simulink model "Quadcopter_Model_V2"  (R2022a)
settings: Solver=ode45  StartTime=0.0  StopTime=20  RelTol=1e-3
values from neighbouring files (symbols this model uses):
  disturbance = false    [Main_Script.m]
  eta = 1    [Linearize_EOM_V2.m]    (also in Properties_Quad.m)
  g = subs(f,x,x_e)    [Linearize_EOM1.m]    (also in Linearize_EOM_V2.m = 9.8; Properties_Quad.m = 9.8)
  L = (F2+F3)*dy - (F1+F4)*dy    [Linearize_EOM1.m]    (also in Linearize_EOM_V2.m = 0.114; Properties_Quad.m = 0.155)
  m = 4    [Controller_LQR.m]    (also in Linearize_EOM1.m; Linearize_EOM_V2.m; Properties_Quad.m = 1)
  noise = false    [Main_Script.m]
  sample = false    [Main_Script.m]
  T = 1-S    [Hinf_Controller_Outer.m]    (also in Properties_Quad.m = 0.01; quad_hinf.m)
  u_e = zeros(4,1)    [A_and_B_Matricies.m]    (also in Controller_LQR.m; Create_System.m; Linear_Main.mat = [2.45 2.45 2.45 2.45]; Linear_Model.mat = [2.45 2.45 2.45 2.45])
undefined symbols (not defined in the file or in its folder): K1, K1_o, K2, K2_o, K3, K3_o
libraries: simulink x2, shared6dof x1
settings Model: Creator=vicen  LastModifiedBy=vicen
settings DebuggingCC: UnconnectedInputMsg=warning  UnconnectedOutputMsg=warning  UnconnectedLineMsg=warning
settings RTWCC: DLArmComputeVersion=19.05

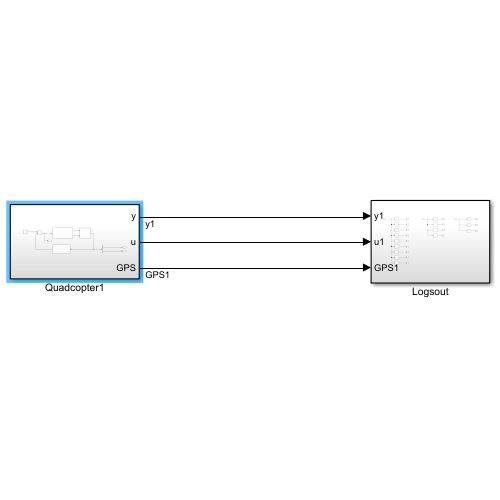
[thumbnail: Simulink's stored preview of the top-level diagram]
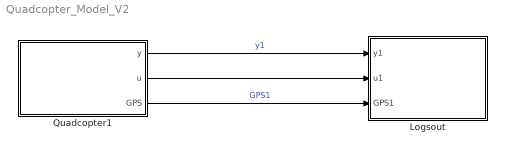
== system Quadcopter_Model_V2 ==
  Logsout : Subsystem
  Quadcopter1 : Subsystem
  wires:
  Quadcopter1/1(y) -> Logsout/1(y1)  "y1"
  Quadcopter1/2(u) -> Logsout/2(u1)
  Quadcopter1/3(GPS) -> Logsout/3(GPS1)  "GPS1"

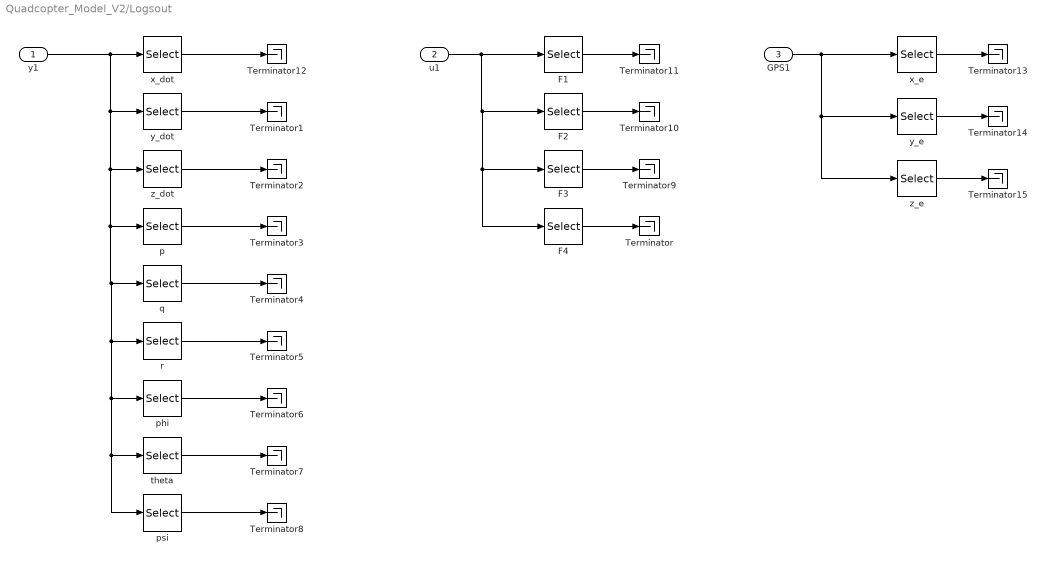
== system Quadcopter_Model_V2/Logsout ==
  y1 : Inport
  u1 : Inport  Port=2
  GPS1 : Inport  Port=3
  F1 : Selector  InputPortWidth=4  IndexOptions=Index vector (dialog)  Indices=1  OutputSizes=1
  F2 : Selector  InputPortWidth=4  IndexOptions=Index vector (dialog)  Indices=2  OutputSizes=1
  F3 : Selector  InputPortWidth=4  IndexOptions=Index vector (dialog)  Indices=3  OutputSizes=1
  F4 : Selector  InputPortWidth=4  IndexOptions=Index vector (dialog)  Indices=4  OutputSizes=1
  Terminator{,1..15} (16 alike) : Terminator
  p : Selector  InputPortWidth=9  IndexOptions=Index vector (dialog)  Indices=4  OutputSizes=1
  phi : Selector  InputPortWidth=9  IndexOptions=Index vector (dialog)  Indices=7  OutputSizes=1
  psi : Selector  InputPortWidth=9  IndexOptions=Index vector (dialog)  Indices=9  OutputSizes=1
  q : Selector  InputPortWidth=9  IndexOptions=Index vector (dialog)  Indices=5  OutputSizes=1
  r : Selector  InputPortWidth=9  IndexOptions=Index vector (dialog)  Indices=6  OutputSizes=1
  theta : Selector  InputPortWidth=9  IndexOptions=Index vector (dialog)  Indices=8  OutputSizes=1
  x_dot : Selector  InputPortWidth=9  IndexOptions=Index vector (dialog)  Indices=1  OutputSizes=1
  x_e : Selector  InputPortWidth=3  IndexOptions=Index vector (dialog)  Indices=1  OutputSizes=1
  y_dot : Selector  InputPortWidth=9  IndexOptions=Index vector (dialog)  Indices=2  OutputSizes=1
  y_e : Selector  InputPortWidth=3  IndexOptions=Index vector (dialog)  Indices=2  OutputSizes=1
  z_dot : Selector  InputPortWidth=9  IndexOptions=Index vector (dialog)  Indices=3  OutputSizes=1
  z_e : Selector  InputPortWidth=3  IndexOptions=Index vector (dialog)  Indices=3  OutputSizes=1
  wires:
  y1/1 -> psi/1, theta/1, phi/1, r/1, q/1, p/1, z_dot/1, y_dot/1, x_dot/1
  x_dot/1 -> Terminator12/1
  y_dot/1 -> Terminator1/1
  z_dot/1 -> Terminator2/1
  p/1 -> Terminator3/1
  q/1 -> Terminator4/1
  r/1 -> Terminator5/1
  phi/1 -> Terminator6/1
  theta/1 -> Terminator7/1
  psi/1 -> Terminator8/1
  u1/1 -> F4/1, F3/1, F2/1, F1/1
  F1/1 -> Terminator11/1
  F2/1 -> Terminator10/1
  F3/1 -> Terminator9/1
  F4/1 -> Terminator/1
  GPS1/1 -> z_e/1, y_e/1, x_e/1
  x_e/1 -> Terminator13/1
  y_e/1 -> Terminator14/1
  z_e/1 -> Terminator15/1

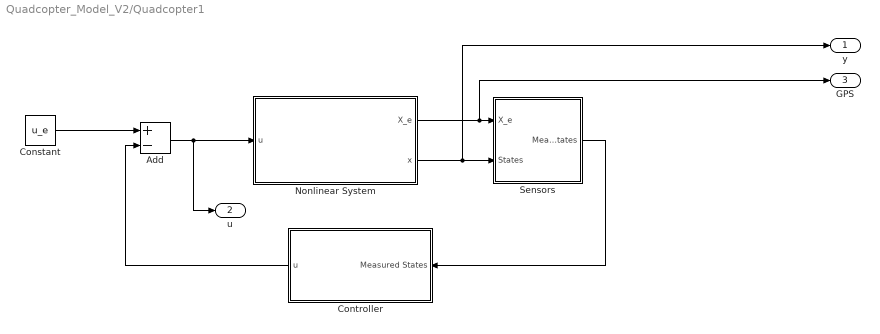
== system Quadcopter_Model_V2/Quadcopter1 ==
  Add : Sum  Inputs=+-
  Constant : Constant  Value=u_e
  Controller : Subsystem
  Nonlinear System : Subsystem
  Sensors : Subsystem
  y : Outport
  u : Outport  Port=2
  GPS : Outport  Port=3
  wires:
  Sensors/1(Measured States) -> Controller/1(Measured States)
  Nonlinear System/1(X_e) -> GPS/1, Sensors/1(X_e)
  Nonlinear System/2(x) -> y/1, Sensors/2(States)
  Controller/1(u) -> Add/2
  Add/1 -> u/1, Nonlinear System/1(u)
  Constant/1 -> Add/1

== system Quadcopter_Model_V2/Quadcopter1/Controller ==
  Measured States : Inport
  Add : Sum
  Inner Loop : Subsystem
  Outer Loop : Subsystem
      settings: PortSchema="{\"entries\":[{\"content\":{\"sides\":[{\"content\":{\"connectorIds\":[\"Out2\",\"Out3\",\"In1\"]},\"type\":\"ConnectorPlacement.EquallySpacedRectSide\",\"uuid\":\"65ae8311-cded-495d-819c-e71778b836d6\"},{\"content\":{\"connectorIds\":[\"Out1\"],\"side\":\"RIGHT\"},\"type\":\"ConnectorPlacement.EquallySpacedRectSide\",\"uuid\":\"cb9e0780-0cb6-488d-9fab-4af44e415d60\"},{\"content\":{\"connectorIds\":[],\"side\":\"TOP\"},\"type\":\"ConnectorPlacement.EquallySpacedRectSide\",\"uuid\":\"e03d7290-0e3a-4bf8-ba18-28e0f329faf8\"}]},\"type\":\"ConnectorPlacement.EquallySpacedConnector\",\"uuid\":\"19cbdee9-600f-46ba-8f26-2065b8c88ffc\"}],\"packageUris\":[\"http://schema.mathworks.com/mf0/Connector/R2020b\"],\"version\":\"1.0\"}"
  u : Outport
  wires:
  Measured States/1 -> Outer Loop/1(Measured States), Inner Loop/1(Measured States)
  Inner Loop/1(u) -> Add/1
  Add/1 -> u/1
  Outer Loop/1(u) -> Add/2
  Outer Loop/3(phi) -> Inner Loop/2(phi)
  Outer Loop/2(theta) -> Inner Loop/3(theta)

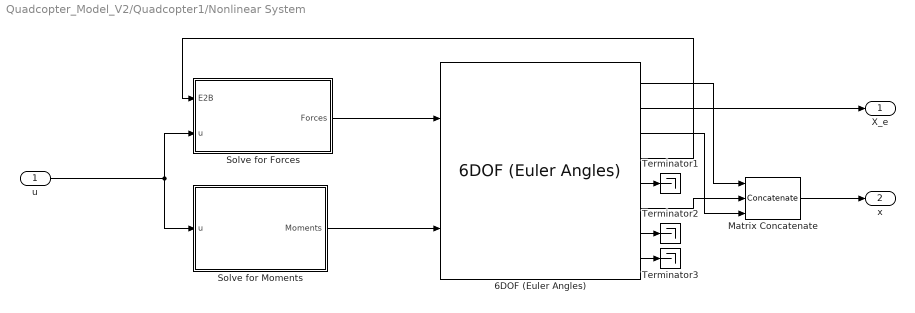
== system Quadcopter_Model_V2/Quadcopter1/Nonlinear System ==
  u : Inport
  6DOF (Euler Angles) : shared6dof/6DOF (Euler Angles)  units=Metric (MKS)  mtype=Fixed  rep=Euler Angles  xme_0=init.pos_e  Vm_0=init.vel_b  eul_0=init.Euler  pm_0=init.rotation_rates_b  mass_0=m  mass_e=0.5  mass_f=2.0  inertia=I  inertia_e=eye(3)  inertia_f=2*eye(3)  k_quat=1.0  vre_flag=on  abi_flag=off  aMode=0  xme_statename=''  Vm_statename=''  eul_statename=''  quat_statename=''  pm_statename=''  mass_statename=''
      settings: SourceProductBaseCode=AE,PW,DR,MT,VE
  Matrix Concatenate : Concatenate  NumInputs=3  ConcatenateDimension=2
  Solve for Forces : Subsystem
  Solve for Moments : Subsystem
  Terminator1 : Terminator
  Terminator2 : Terminator
  Terminator3 : Terminator
  X_e : Outport
  x : Outport  Port=2
  wires:
  6DOF (Euler Angles)/8 -> Terminator3/1
  6DOF (Euler Angles)/1 -> Matrix Concatenate/1
  6DOF (Euler Angles)/7 -> Terminator2/1
  u/1 -> Solve for Moments/1(u), Solve for Forces/2(u)
  6DOF (Euler Angles)/6 -> Matrix Concatenate/2
  6DOF (Euler Angles)/3 -> Matrix Concatenate/3
  6DOF (Euler Angles)/5 -> Terminator1/1
  Solve for Moments/1(Moments) -> 6DOF (Euler Angles)/2
  6DOF (Euler Angles)/2 -> X_e/1
  Matrix Concatenate/1 -> x/1
  Solve for Forces/1(Forces) -> 6DOF (Euler Angles)/1
  6DOF (Euler Angles)/4 -> Solve for Forces/1(E2B)

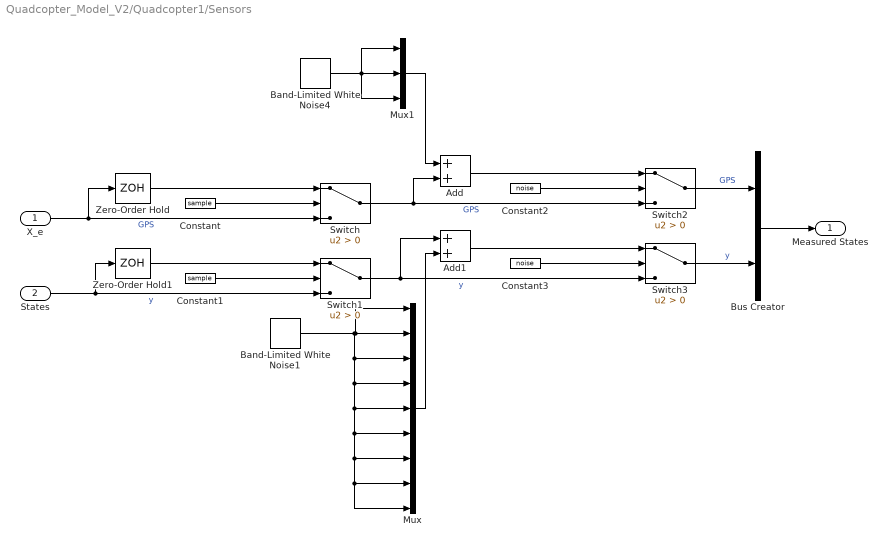
== system Quadcopter_Model_V2/Quadcopter1/Sensors ==
  X_e : Inport
  States : Inport  Port=2
  Add : Sum
  Add1 : Sum
  Band-Limited White Noise1 : simulink/Sources/Band-Limited White Noise  Cov=[0.00001]  Ts=0.01  seed=[23341]
  Band-Limited White Noise4 : simulink/Sources/Band-Limited White Noise  Cov=[0.00001]  Ts=0.01  seed=[23341]
  Bus Creator : BusCreator  Inputs=2
  Constant : Constant  Value=sample
  Constant1 : Constant  Value=sample
  Constant2 : Constant  Value=noise
  Constant3 : Constant  Value=noise
  Mux : Mux  Inputs=9
  Mux1 : Mux  Inputs=3
  Switch{,1..3} (4 alike) : Switch  Criteria=u2 > Threshold  SaturateOnIntegerOverflow=off  InputSameDT=off
  Zero-Order Hold : ZeroOrderHold  SampleTime=T
  Zero-Order Hold1 : ZeroOrderHold  SampleTime=T
  Measured States : Outport
  wires:
  States/1 -> Zero-Order Hold1/1, Switch1/3  "y"
  Bus Creator/1 -> Measured States/1
  X_e/1 -> Switch/3, Zero-Order Hold/1  "GPS"
  Constant/1 -> Switch/2
  Constant1/1 -> Switch1/2
  Zero-Order Hold/1 -> Switch/1
  Zero-Order Hold1/1 -> Switch1/1
  Switch2/1 -> Bus Creator/1  "GPS"
  Switch3/1 -> Bus Creator/2  "y"
  Add1/1 -> Switch3/1
  Add/1 -> Switch2/1
  Constant3/1 -> Switch3/2
  Constant2/1 -> Switch2/2
  Switch/1 -> Add/2, Switch2/3  "GPS"
  Switch1/1 -> Add1/1, Switch3/3  "y"
  Band-Limited White Noise1/1 -> Mux/2, Mux/1, Mux/3, Mux/4, Mux/6, Mux/8, Mux/9, Mux/7, Mux/5
  Mux/1 -> Add1/2
  Mux1/1 -> Add/1
  Band-Limited White Noise4/1 -> Mux1/1, Mux1/2, Mux1/3

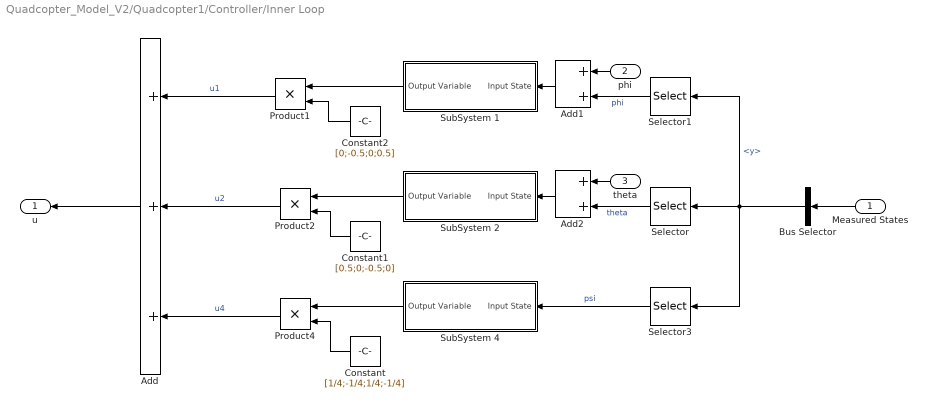
== system Quadcopter_Model_V2/Quadcopter1/Controller/Inner Loop ==
  Measured States : Inport
  phi : Inport  Port=2
  theta : Inport  Port=3
  Add : Sum  Inputs=+++
  Add1 : Sum
  Add2 : Sum
  Bus Selector : BusSelector  OutputSignals=y
  Constant : Constant  Value=[1/4;-1/4;1/4;-1/4]
  Constant1 : Constant  Value=[0.5;0;-0.5;0]
  Constant2 : Constant  Value=[0;-0.5;0;0.5]
  Product1 : Product
  Product2 : Product
  Product4 : Product
  Selector : Selector  InputPortWidth=9  IndexOptions=Index vector (dialog)  Indices=8  OutputSizes=1
  Selector1 : Selector  InputPortWidth=9  IndexOptions=Index vector (dialog)  Indices=7  OutputSizes=1
  Selector3 : Selector  InputPortWidth=9  IndexOptions=Index vector (dialog)  Indices=9  OutputSizes=1
  SubSystem 1 : Subsystem
  SubSystem 2 : Subsystem
  SubSystem 4 : Subsystem
  u : Outport
  wires:
  Constant2/1 -> Product1/2
  Bus Selector/1 -> Selector1/1, Selector3/1, Selector/1  "<y>"
  Product2/1 -> Add/2  "u2"
  Selector1/1 -> Add1/2  "phi"
  SubSystem 1/1(Output Variable) -> Product1/1
  Product1/1 -> Add/1  "u1"
  Selector/1 -> Add2/2  "theta"
  Measured States/1 -> Bus Selector/1
  Constant1/1 -> Product2/2
  SubSystem 4/1(Output Variable) -> Product4/1
  Constant/1 -> Product4/2
  Product4/1 -> Add/3  "u4"
  SubSystem 2/1(Output Variable) -> Product2/1
  Selector3/1 -> SubSystem 4/1(Input State)  "psi"
  Add/1 -> u/1
  Add1/1 -> SubSystem 1/1(Input State)
  Add2/1 -> SubSystem 2/1(Input State)
  phi/1 -> Add1/1
  theta/1 -> Add2/1

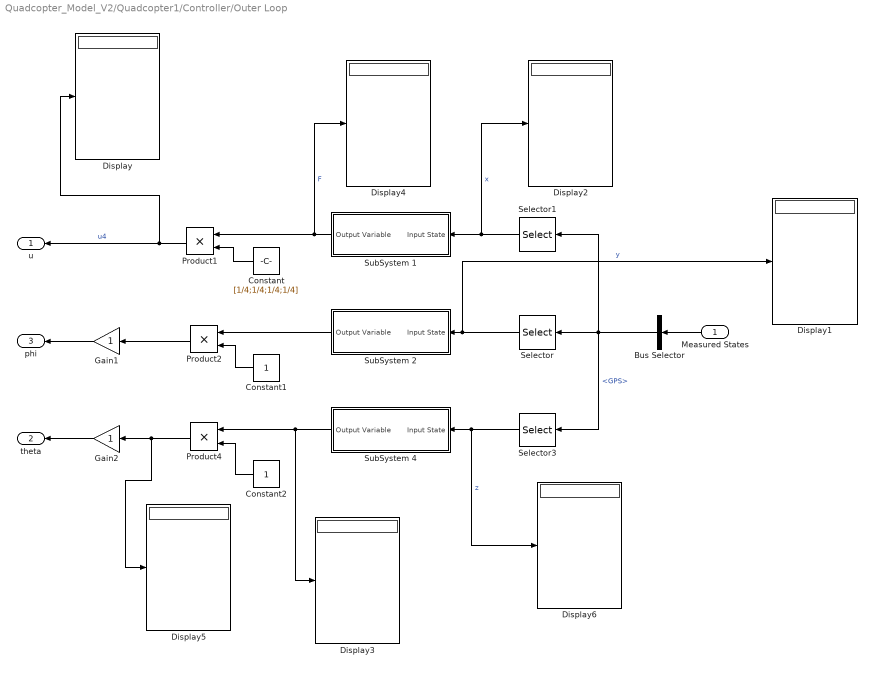
== system Quadcopter_Model_V2/Quadcopter1/Controller/Outer Loop ==
  Measured States : Inport
  Bus Selector : BusSelector  OutputSignals=GPS
  Constant : Constant  Value=[1/4;1/4;1/4;1/4]
  Constant1 : Constant
  Constant2 : Constant
  Display{,1..6} (7 alike) : Display
  Gain1 : Gain
  Gain2 : Gain
  Product1 : Product
  Product2 : Product
  Product4 : Product
  Selector : Selector  InputPortWidth=3  IndexOptions=Index vector (dialog)  Indices=2  OutputSizes=1
  Selector1 : Selector  InputPortWidth=3  IndexOptions=Index vector (dialog)  Indices=3  OutputSizes=1
  Selector3 : Selector  InputPortWidth=3  IndexOptions=Index vector (dialog)  Indices=1  OutputSizes=1
  SubSystem 1 : Subsystem
  SubSystem 2 : Subsystem
  SubSystem 4 : Subsystem
  u : Outport
  theta : Outport  Port=2
  phi : Outport  Port=3
  wires:
  Selector3/1 -> Display6/1, SubSystem 4/1(Input State)  "z"
  SubSystem 2/1(Output Variable) -> Product2/1
  Constant/1 -> Product1/2
  SubSystem 4/1(Output Variable) -> Product4/1, Display3/1
  Constant1/1 -> Product2/2
  Measured States/1 -> Bus Selector/1
  Selector/1 -> SubSystem 2/1(Input State), Display1/1  "y"
  Product1/1 -> u/1, Display/1  "u4"
  SubSystem 1/1(Output Variable) -> Display4/1, Product1/1  "F"
  Selector1/1 -> Display2/1, SubSystem 1/1(Input State)  "x"
  Bus Selector/1 -> Selector/1, Selector1/1, Selector3/1  "<GPS>"
  Constant2/1 -> Product4/2
  Product2/1 -> Gain1/1
  Product4/1 -> Gain2/1, Display5/1
  Gain1/1 -> phi/1
  Gain2/1 -> theta/1

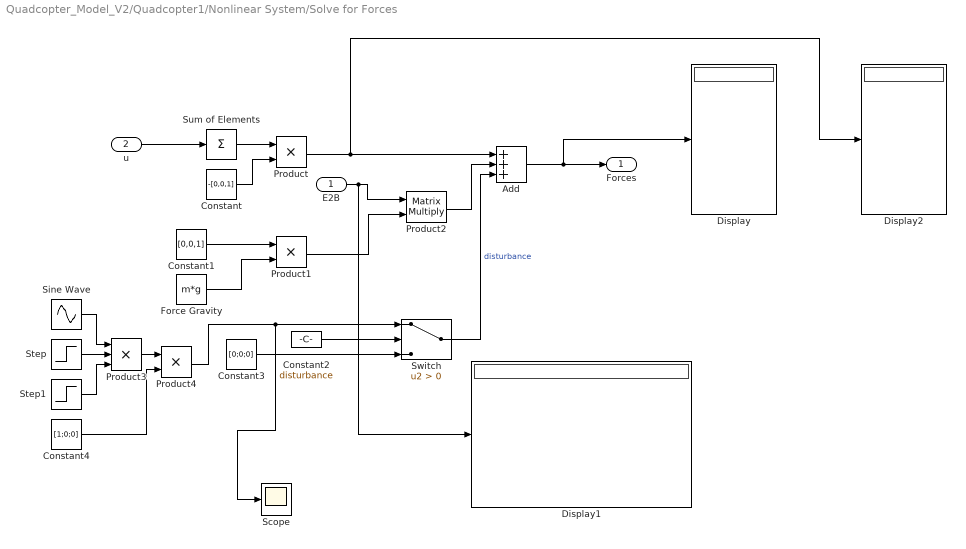
== system Quadcopter_Model_V2/Quadcopter1/Nonlinear System/Solve for Forces ==
  E2B : Inport
  u : Inport  Port=2
  Add : Sum  Inputs=+++
  Constant : Constant  Value=-[0,0,1]
  Constant1 : Constant  Value=[0,0,1]
  Constant2 : Constant  Value=disturbance
  Constant3 : Constant  Value=[0;0;0]
  Constant4 : Constant  Value=[1;0;0]
  Display : Display
  Display1 : Display
  Display2 : Display
  Force Gravity : Constant  Value=m*g
  Product : Product
  Product1 : Product
  Product2 : Product  Multiplication=Matrix(*)
  Product3 : Product  Inputs=3
  Product4 : Product
  Scope : Scope
  Sine Wave : Sin  Amplitude=0.1149  Frequency=pi/5  Phase=pi  SampleTime=0
  Step : Step  Time=5  SampleTime=0
  Step1 : Step  Time=10  Before=1  After=0  SampleTime=0
  Sum of Elements : Sum  Inputs=+
  Switch : Switch  Criteria=u2 > Threshold  SaturateOnIntegerOverflow=off  InputSameDT=off
  Forces : Outport
  wires:
  Product1/1 -> Product2/2
  Product2/1 -> Add/2
  Force Gravity/1 -> Product1/2
  Product/1 -> Display2/1, Add/1
  Constant1/1 -> Product1/1
  Constant/1 -> Product/2
  Sum of Elements/1 -> Product/1
  Add/1 -> Display/1, Forces/1
  u/1 -> Sum of Elements/1
  E2B/1 -> Display1/1, Product2/1
  Switch/1 -> Add/3  "disturbance"
  Constant2/1 -> Switch/2
  Constant3/1 -> Switch/3
  Sine Wave/1 -> Product3/1
  Step/1 -> Product3/2
  Product3/1 -> Product4/1
  Constant4/1 -> Product4/2
  Product4/1 -> Scope/1, Switch/1
  Step1/1 -> Product3/3

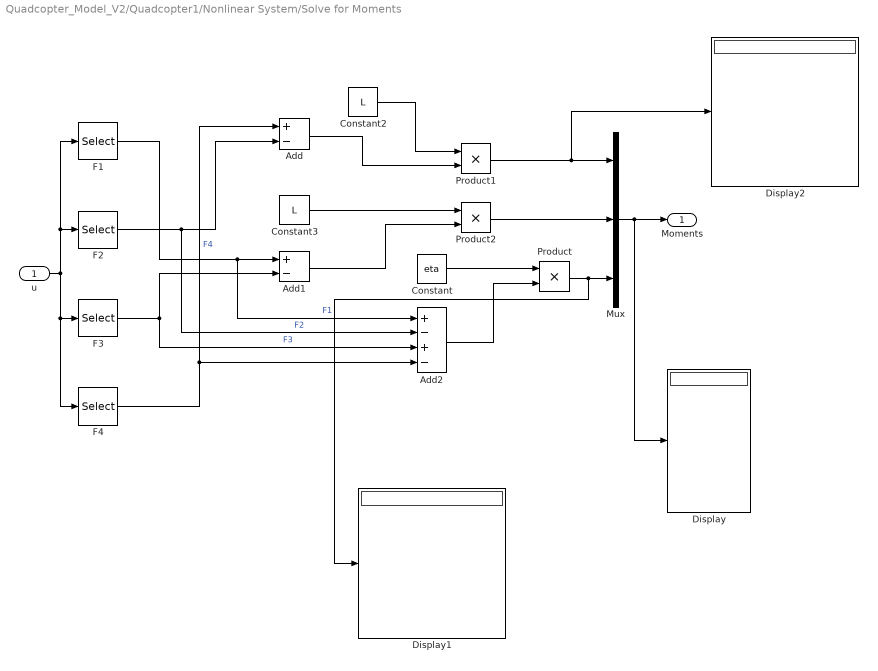
== system Quadcopter_Model_V2/Quadcopter1/Nonlinear System/Solve for Moments ==
  u : Inport
  Add : Sum  Inputs=+-
  Add1 : Sum  Inputs=+-
  Add2 : Sum  Inputs=+-+-
  Constant : Constant  Value=eta
  Constant2 : Constant  Value=L
  Constant3 : Constant  Value=L
  Display : Display
  Display1 : Display
  Display2 : Display
  F1 : Selector  InputPortWidth=4  IndexOptions=Index vector (dialog)  Indices=1  OutputSizes=1
  F2 : Selector  InputPortWidth=4  IndexOptions=Index vector (dialog)  Indices=2  OutputSizes=1
  F3 : Selector  InputPortWidth=4  IndexOptions=Index vector (dialog)  Indices=3  OutputSizes=1
  F4 : Selector  InputPortWidth=4  IndexOptions=Index vector (dialog)  Indices=4  OutputSizes=1
  Mux : Mux  Inputs=3
  Product : Product
  Product1 : Product
  Product2 : Product
  Moments : Outport
  wires:
  Mux/1 -> Display/1, Moments/1
  u/1 -> F1/1, F2/1, F4/1, F3/1
  F2/1 -> Add2/2, Add/2  "F2"
  F3/1 -> Add2/3, Add1/2  "F3"
  F4/1 -> Add2/4, Add/1  "F4"
  Constant/1 -> Product/1
  Constant2/1 -> Product1/1
  Product1/1 -> Display2/1, Mux/1
  Product2/1 -> Mux/2
  Constant3/1 -> Product2/1
  Add/1 -> Product1/2
  Add1/1 -> Product2/2
  F1/1 -> Add2/1, Add1/1  "F1"
  Product/1 -> Display1/1, Mux/3
  Add2/1 -> Product/2

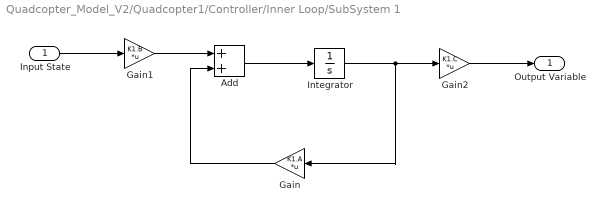
== system Quadcopter_Model_V2/Quadcopter1/Controller/Inner Loop/SubSystem 1 ==
  Input State : Inport
  Add : Sum
  Gain : Gain  Gain=K1.A  Multiplication=Matrix(K*u)
  Gain1 : Gain  Gain=K1.B  Multiplication=Matrix(K*u)
  Gain2 : Gain  Gain=K1.C  Multiplication=Matrix(K*u)
  Integrator : Integrator
  Output Variable : Outport
  wires:
  Input State/1 -> Gain1/1
  Gain1/1 -> Add/1
  Add/1 -> Integrator/1
  Integrator/1 -> Gain2/1, Gain/1
  Gain/1 -> Add/2
  Gain2/1 -> Output Variable/1

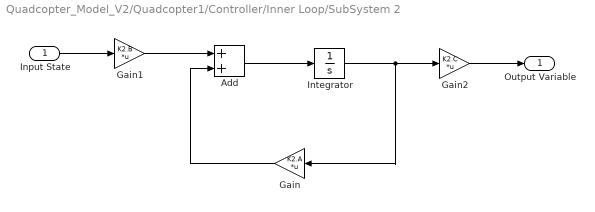
== system Quadcopter_Model_V2/Quadcopter1/Controller/Inner Loop/SubSystem 2 ==
  Input State : Inport
  Add : Sum
  Gain : Gain  Gain=K2.A  Multiplication=Matrix(K*u)
  Gain1 : Gain  Gain=K2.B  Multiplication=Matrix(K*u)
  Gain2 : Gain  Gain=K2.C  Multiplication=Matrix(K*u)
  Integrator : Integrator
  Output Variable : Outport
  wires:
  Gain/1 -> Add/2
  Integrator/1 -> Gain/1, Gain2/1
  Add/1 -> Integrator/1
  Gain1/1 -> Add/1
  Input State/1 -> Gain1/1
  Gain2/1 -> Output Variable/1

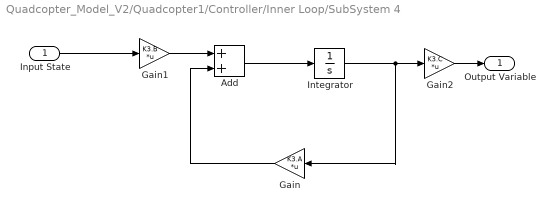
== system Quadcopter_Model_V2/Quadcopter1/Controller/Inner Loop/SubSystem 4 ==
  Input State : Inport
  Add : Sum
  Gain : Gain  Gain=K3.A  Multiplication=Matrix(K*u)
  Gain1 : Gain  Gain=K3.B  Multiplication=Matrix(K*u)
  Gain2 : Gain  Gain=K3.C  Multiplication=Matrix(K*u)
  Integrator : Integrator
  Output Variable : Outport
  wires:
  Gain/1 -> Add/2
  Integrator/1 -> Gain/1, Gain2/1
  Add/1 -> Integrator/1
  Gain1/1 -> Add/1
  Input State/1 -> Gain1/1
  Gain2/1 -> Output Variable/1

== system Quadcopter_Model_V2/Quadcopter1/Controller/Outer Loop/SubSystem 1 ==
  Input State : Inport
  Add : Sum
  Gain : Gain  Gain=K3_o.A  Multiplication=Matrix(K*u)
  Gain1 : Gain  Gain=K3_o.B  Multiplication=Matrix(K*u)
  Gain2 : Gain  Gain=K3_o.C  Multiplication=Matrix(K*u)
  Integrator : Integrator
  Output Variable : Outport
  wires:
  Gain2/1 -> Output Variable/1
  Gain/1 -> Add/2
  Integrator/1 -> Gain/1, Gain2/1
  Add/1 -> Integrator/1
  Gain1/1 -> Add/1
  Input State/1 -> Gain1/1

== system Quadcopter_Model_V2/Quadcopter1/Controller/Outer Loop/SubSystem 2 ==
  Input State : Inport
  Add : Sum
  Gain : Gain  Gain=K2_o.A  Multiplication=Matrix(K*u)
  Gain1 : Gain  Gain=K2_o.B  Multiplication=Matrix(K*u)
  Gain2 : Gain  Gain=K2_o.C  Multiplication=Matrix(K*u)
  Integrator : Integrator
  Output Variable : Outport
  wires:
  Gain2/1 -> Output Variable/1
  Input State/1 -> Gain1/1
  Gain1/1 -> Add/1
  Add/1 -> Integrator/1
  Integrator/1 -> Gain2/1, Gain/1
  Gain/1 -> Add/2

== system Quadcopter_Model_V2/Quadcopter1/Controller/Outer Loop/SubSystem 4 ==
  Input State : Inport
  Add : Sum
  Gain : Gain  Gain=K1_o.A  Multiplication=Matrix(K*u)
  Gain1 : Gain  Gain=K1_o.B  Multiplication=Matrix(K*u)
  Gain2 : Gain  Gain=K1_o.C  Multiplication=Matrix(K*u)
  Integrator : Integrator
  Output Variable : Outport
  wires:
  Gain2/1 -> Output Variable/1
  Input State/1 -> Gain1/1
  Gain1/1 -> Add/1
  Add/1 -> Integrator/1
  Integrator/1 -> Gain2/1, Gain/1
  Gain/1 -> Add/2
